simulink model "TDoFs_mass_CL_Trajopt"  (R2022b)
settings: Solver=FixedStepAuto  StartTime=0.0  StopTime=10.0  FixedStep=0.0001  RelTol=1e-3
settings Model: Creator=Taehoon Kim  LastModifiedBy=User
settings ModelReferenceCC: EnableRefExpFcnMdlSchedulingChecks=on

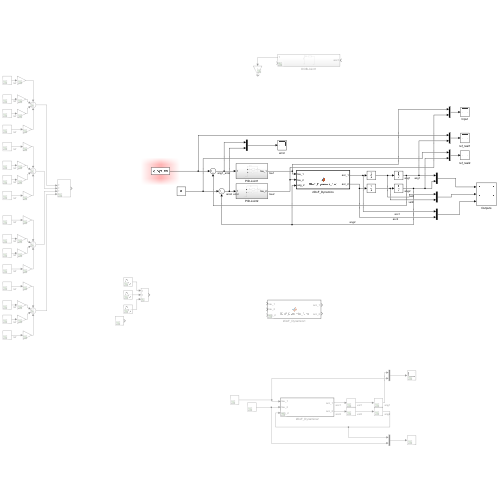
[thumbnail: Simulink's stored preview of the top-level diagram]
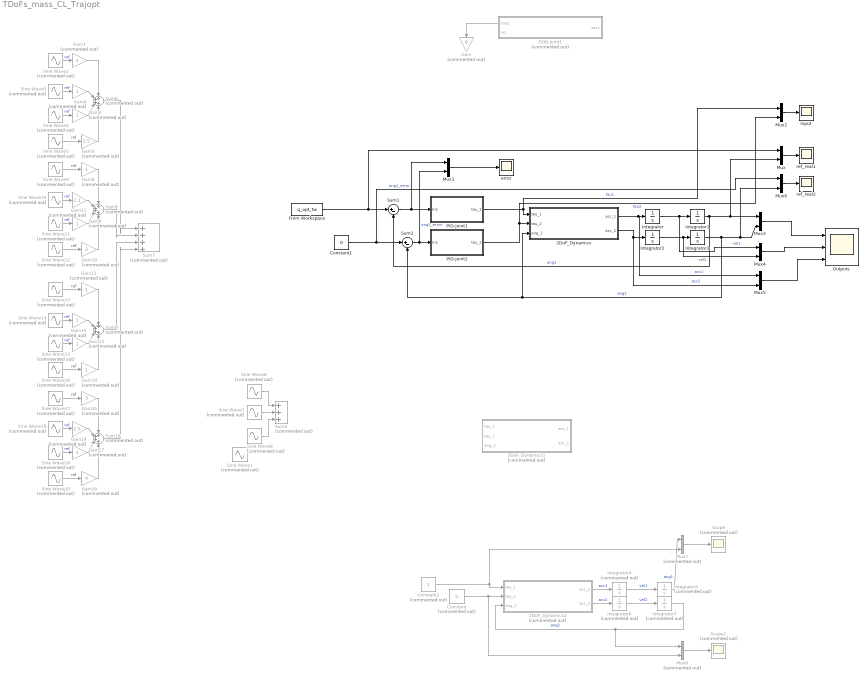
== system TDoFs_mass_CL_Trajopt ==
  2DoF_Dynamics : MATLAB Function  TreatAsAtomicUnit=on
  2DoF_Dynamics1 : MATLAB Function  Commented=on  TreatAsAtomicUnit=on
  2DoF_Dynamics2 : MATLAB Function  Commented=on  TreatAsAtomicUnit=on
  Constant : Constant  Commented=on  Value=0
  Constant1 : Constant  Value=0
  Constant2 : Constant  Commented=on
  DOB-Joint1 : Subsystem  Commented=on
      settings: PortSchema="{\"entries\":[{\"content\":{\"sides\":[{\"content\":{\"connectorIds\":[\"Out1\",\"In1\"]},\"type\":\"ConnectorPlacement.EquallySpacedRectSide\",\"uuid\":\"aed64ee6-890a-40cf-96da-aa5fbca5e20d\"},{\"content\":{\"connectorIds\":[\"In2\"],\"side\":\"RIGHT\"},\"type\":\"ConnectorPlacement.EquallySpacedRectSide\",\"uuid\":\"6cb1d59b-7b2e-4e62-91b9-34dc0f1a000d\"},{\"content\":{\"connectorIds\":[],\"side\":\"TOP\"},\"type\":\"ConnectorPlacement.EquallySpacedRectSide\",\"uuid\":\"fc023f32-e7f5-4e50-b17a-39a9cd0cd429\"},{\"content\":{\"connectorIds\":[],\"side\":\"BOTTOM\"},\"type\":\"ConnectorPlacement.EquallySpacedRectSide\",\"uuid\":\"89f43edb-87a0-44d2-8db4-1bc101ff0a7e\"}]},\"type\":\"ConnectorPlacement.EquallySpacedConnector\",\"uuid\":\"a2668ce1-ca6b-486c-8b99-a7467b774e8d\"}],\"packageUris\":[\"http://schema.mathworks.com/mf0/Connector/R2020b\"],\"version\":\"1.0\"}"
  From Workspace : FromWorkspace  VariableName=q_opt_tw  OutDataTypeStr=double  SampleTime=0.001
  Gain : Gain  Commented=on  Gain=0
  Gain1 : Gain  Commented=on  Gain=5
  Gain10 : Gain  Commented=on  Gain=2
  Gain11 : Gain  Commented=on  Gain=2.1
  Gain{2,4,8..9,12..15,17} (9 alike) : Gain  Commented=on
  Gain16 : Gain  Commented=on  Gain=3
  Gain18 : Gain  Commented=on  Gain=4
  Gain19 : Gain  Commented=on  Gain=2.5
  Gain3 : Gain  Commented=on  Gain=1.5
  Input : Scope
  Integrator{,1..3} (4 alike) : Integrator
  Integrator{4..7} (4 alike) : Integrator  Commented=on
  Mux{,1..6} (7 alike) : Mux  Inputs=2
  Mux7 : Mux  Commented=on  Inputs=2
  Mux8 : Mux  Commented=on  Inputs=2
  Outputs : Scope  NumInputPorts=3
  PID-Joint1 : Subsystem
  PID-Joint2 : Subsystem
  Scope : Scope  Commented=on
  Scope1 : Scope  Commented=on
  Sine Wave1 : Sin  Commented=on  Amplitude=30*(pi/180)  Frequency=2*pi*0.5  SampleTime=0
  Sine Wave10 : Sin  Commented=on  Amplitude=1*(pi/180)  Frequency=0.6*2*pi  SampleTime=0
  Sine Wave11 : Sin  Commented=on  Amplitude=2.1*(pi/180)  Frequency=0.7*2*pi  SampleTime=0
  Sine Wave12 : Sin  Commented=on  Amplitude=2.2*(pi/180)  Frequency=0.8*2*pi  SampleTime=0
  Sine Wave13 : Sin  Commented=on  Amplitude=2*(pi/180)  Frequency=0.9*2*pi  SampleTime=0
  Sine Wave14 : Sin  Commented=on  Amplitude=1.9*(pi/180)  Frequency=1*2*pi  SampleTime=0
  Sine Wave15 : Sin  Commented=on  Amplitude=1.8*(pi/180)  Frequency=1.1*2*pi  SampleTime=0
  Sine Wave16 : Sin  Commented=on  Amplitude=1.7*(pi/180)  Frequency=1.2*2*pi  SampleTime=0
  Sine Wave17 : Sin  Commented=on  Amplitude=1.6*(pi/180)  Frequency=1.3*2*pi  SampleTime=0
  Sine Wave18 : Sin  Commented=on  Amplitude=1.5*(pi/180)  Frequency=1.4*2*pi  SampleTime=0
  Sine Wave19 : Sin  Commented=on  Amplitude=1.3*(pi/180)  Frequency=1.5*2*pi  SampleTime=0
  Sine Wave2 : Sin  Commented=on  Amplitude=1*(pi/180)  Frequency=0.1*2*pi  SampleTime=0
  Sine Wave20 : Sin  Commented=on  Amplitude=1.2*(pi/180)  Frequency=1.5*2*pi  SampleTime=0
  Sine Wave3 : Sin  Commented=on  Amplitude=1.1*(pi/180)  Frequency=0.2*2*pi  SampleTime=0
  Sine Wave4 : Sin  Commented=on  Amplitude=2.4*(pi/180)  Frequency=0.3*2*pi  SampleTime=0
  Sine Wave5 : Sin  Commented=on  Amplitude=2.5*(pi/180)  Frequency=0.4*2*pi  SampleTime=0
  Sine Wave6 : Sin  Commented=on  Amplitude=10*(pi/180)  Frequency=1*2*pi  SampleTime=0
  Sine Wave7 : Sin  Commented=on  Amplitude=20*(pi/180)  Frequency=0.8*2*pi  SampleTime=0
  Sine Wave8 : Sin  Commented=on  Amplitude=2*(pi/180)  Frequency=0.5*2*pi  SampleTime=0
  Sine Wave9 : Sin  Commented=on  Amplitude=2.3*(pi/180)  Frequency=0.5*2*pi  SampleTime=0
  Sum1 : Sum  Inputs=|+-
  Sum{6,8..10} (4 alike) : Sum  Commented=on  Inputs=++++
  Sum2 : Sum  Inputs=|+-
  Sum4 : Sum  Commented=on  Inputs=+++
  Sum7 : Sum  Commented=on  Inputs=|++++
  error : Scope
  ref_real1 : Scope
  ref_real2 : Scope
  wires:
  Integrator1/1 -> Mux/2, Mux3/1, Sum1/2  "ang1"
  Integrator/1 -> Integrator1/1, Mux4/1  "vel1"
  Mux/1 -> ref_real1/1
  Sum1/1 -> Mux1/1, PID-Joint1/1(In1)  "ang1_error"
  PID-Joint1/1(tau_1) -> 2DoF_Dynamics/1(tau_1), Mux2/1  "tau1"
  PID-Joint2/1(tau_2) -> 2DoF_Dynamics/2(tau_2), Mux2/2  "tau2"
  Sum2/1 -> Mux1/2, PID-Joint2/1(In1)  "ang2_error"
  Mux1/1 -> error/1
  Mux2/1 -> Input/1
  2DoF_Dynamics/2(acc_2) -> Integrator2/1, Mux5/2  "acc2"
  Integrator2/1 -> Integrator3/1, Mux4/2  "vel2"
  Integrator3/1 -> Sum2/2, 2DoF_Dynamics/3(ang_2), Mux6/2, Mux3/2  "ang2"
  Mux3/1 -> Outputs/1
  Mux4/1 -> Outputs/2
  2DoF_Dynamics/1(acc_1) -> Mux5/1, Integrator/1  "acc1"
  Mux5/1 -> Outputs/3
  Mux6/1 -> ref_real2/1
  Constant2/1 -> 2DoF_Dynamics2/1(tau_1), Mux7/2
  Constant/1 -> Mux8/2, 2DoF_Dynamics2/2(tau_2)
  2DoF_Dynamics2/1(acc_1) -> Integrator4/1  "acc1"
  Integrator4/1 -> Integrator5/1  "vel1"
  2DoF_Dynamics2/2(acc_2) -> Integrator6/1  "acc2"
  Integrator6/1 -> Integrator7/1  "vel2"
  Integrator7/1 -> Mux8/1, 2DoF_Dynamics2/3(ang_2)  "ang2"
  Integrator5/1 -> Mux7/1  "ang1"
  Mux7/1 -> Scope/1
  Mux8/1 -> Scope1/1
  DOB-Joint1/1(Out1) -> Gain/1
  Sum8/1 -> Sum7/2
  Sine Wave13/1 -> Gain12/1  "ref"
  Sine Wave15/1 -> Gain13/1  "ref"
  Gain15/1 -> Sum9/2
  Gain9/1 -> Sum8/3
  Sine Wave19/1 -> Gain17/1  "ref"
  Gain11/1 -> Sum8/2
  Sum9/1 -> Sum7/3
  Gain14/1 -> Sum9/4
  Sine Wave12/1 -> Gain10/1  "ref"
  Sine Wave20/1 -> Gain18/1  "ref"
  Gain10/1 -> Sum8/4
  Gain3/1 -> Sum6/4
  Sine Wave14/1 -> Gain15/1  "ref"
  Gain18/1 -> Sum10/4
  Gain16/1 -> Sum10/1
  Gain17/1 -> Sum10/3
  Sine Wave10/1 -> Gain11/1  "ref"
  Sum10/1 -> Sum7/4
  Gain2/1 -> Sum6/3
  Sine Wave18/1 -> Gain19/1  "ref"
  Gain4/1 -> Sum6/2
  Sine Wave17/1 -> Gain16/1  "ref"
  Gain19/1 -> Sum10/2
  Gain13/1 -> Sum9/3
  Sine Wave3/1 -> Gain4/1  "ref"
  Sine Wave11/1 -> Gain9/1  "ref"
  Gain12/1 -> Sum9/1
  Sine Wave16/1 -> Gain14/1  "ref"
  Sine Wave4/1 -> Gain2/1  "ref"
  Gain8/1 -> Sum8/1
  Sum6/1 -> Sum7/1
  Sine Wave9/1 -> Gain8/1  "ref"
  Sine Wave5/1 -> Gain3/1  "ref"
  Gain1/1 -> Sum6/1
  Sine Wave2/1 -> Gain1/1  "ref"
  From Workspace/1 -> Mux/1, Sum1/1
  Sine Wave6/1 -> Sum4/1
  Sine Wave8/1 -> Sum4/3
  Sine Wave7/1 -> Sum4/2
  Constant1/1 -> Mux6/1, Sum2/1

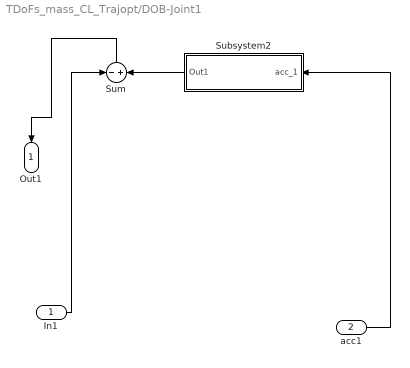
== system TDoFs_mass_CL_Trajopt/DOB-Joint1 ==
  In1 : Inport
  acc1 : Inport  Port=2
  Subsystem2 : Subsystem
  Sum : Sum  Inputs=-+
  Out1 : Outport
  wires:
  In1/1 -> Sum/1
  acc1/1 -> Subsystem2/1(acc_1)
  Subsystem2/1(Out1) -> Sum/2
  Sum/1 -> Out1/1

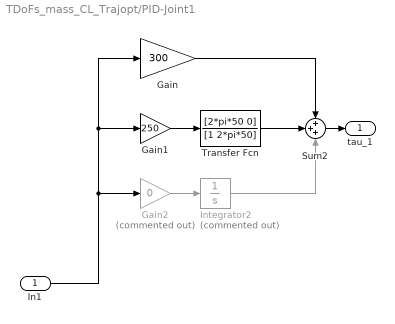
== system TDoFs_mass_CL_Trajopt/PID-Joint1 ==
  In1 : Inport
  Gain : Gain  Gain=300
  Gain1 : Gain  Gain=250
  Gain2 : Gain  Commented=on  Gain=0
  Integrator2 : Integrator  Commented=on
  Sum2 : Sum  Inputs=+++
  Transfer Fcn : TransferFcn  Numerator=[2*pi*50 0]  Denominator=[1 2*pi*50]
  tau_1 : Outport
  wires:
  Gain1/1 -> Transfer Fcn/1
  Gain/1 -> Sum2/1
  Integrator2/1 -> Sum2/3
  In1/1 -> Gain2/1, Gain/1, Gain1/1
  Transfer Fcn/1 -> Sum2/2
  Gain2/1 -> Integrator2/1
  Sum2/1 -> tau_1/1

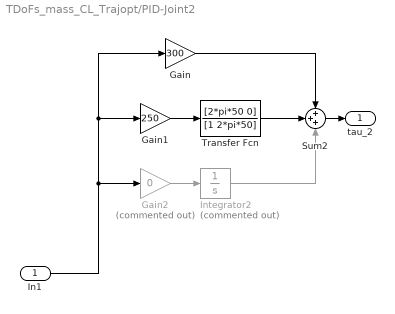
== system TDoFs_mass_CL_Trajopt/PID-Joint2 ==
  In1 : Inport
  Gain : Gain  Gain=300
  Gain1 : Gain  Gain=250
  Gain2 : Gain  Commented=on  Gain=0
  Integrator2 : Integrator  Commented=on
  Sum2 : Sum  Inputs=+++
  Transfer Fcn : TransferFcn  Numerator=[2*pi*50 0]  Denominator=[1 2*pi*50]
  tau_2 : Outport
  wires:
  Sum2/1 -> tau_2/1
  Gain2/1 -> Integrator2/1
  Transfer Fcn/1 -> Sum2/2
  In1/1 -> Gain1/1, Gain/1, Gain2/1
  Integrator2/1 -> Sum2/3
  Gain/1 -> Sum2/1
  Gain1/1 -> Transfer Fcn/1

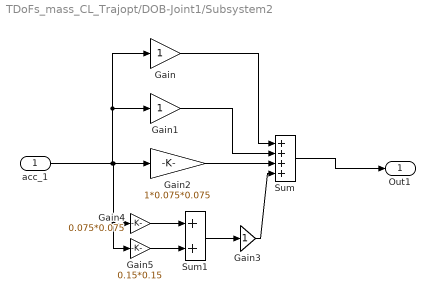
== system TDoFs_mass_CL_Trajopt/DOB-Joint1/Subsystem2 ==
  acc_1 : Inport
  Gain : Gain
  Gain1 : Gain
  Gain2 : Gain  Gain=1*0.075*0.075
  Gain3 : Gain
  Gain4 : Gain  Gain=0.075*0.075
  Gain5 : Gain  Gain=0.15*0.15
  Sum : Sum  Inputs=++++
  Sum1 : Sum
  Out1 : Outport
  wires:
  Sum/1 -> Out1/1
  Gain2/1 -> Sum/3
  Gain1/1 -> Sum/2
  Gain/1 -> Sum/1
  acc_1/1 -> Gain/1, Gain1/1, Gain5/1, Gain4/1, Gain2/1
  Gain3/1 -> Sum/4
  Sum1/1 -> Gain3/1
  Gain4/1 -> Sum1/1
  Gain5/1 -> Sum1/2

== matlab function TDoFs_mass_CL_Trajopt/2DoF_Dynamics1 ==
  data: tau_1 input; acc_1 output; tau_2 input; ang_2 input; acc_2 output
function [acc_1, acc_2] = TDoF_Dynamics_func(tau_1, tau_2, ang_2)
    % Parameters
    J1 = 1;
    J2 = 1;
    l1 = 0.15;
    m2 = 1;
    d1 = 0.075;
    d2 = 0.075;
    
    D = (J2+m2*d2^2)*(J1+J2+m2*d1^2+m2*(2*l1*d2*cos(ang_2)+l1^2+d2^2))-(J2+m2*(l1*d2*cos(ang_2)+d2^2))^2;
    
    acc_1 = ((J2+m2*d2^2)*tau_1+(-J2-m2*(l1*d2*cos(ang_2)+d2^2))*tau_2)/D;
    acc_2 = ((-J2-m2*(l1*d2*cos(ang_2)+d2^2))*tau_1+(J1+J2+m2*d1^2+m2*(2*l1*d2*cos(ang_2)+l1^2+d2^2))*tau_2)/D;
end

== matlab function TDoFs_mass_CL_Trajopt/2DoF_Dynamics ==
  data: tau_1 input; acc_1 output; tau_2 input; ang_2 input; acc_2 output
function [acc_1, acc_2] = TDoF_Dynamics_func(tau_1, tau_2, ang_2)
    % Parameters
    J1 = 1;
    J2 = 1;
    l1 = 0.15;
    m2 = 1;
    d1 = 0.075;
    d2 = 0.075;
    
    D = (J2+m2*d2^2)*(J1+J2+m2*d1^2+m2*(2*l1*d2*cos(ang_2)+l1^2+d2^2))-(J2+m2*(l1*d2*cos(ang_2)+d2^2))^2;
    
    acc_1 = ((J2+m2*d2^2)*tau_1+(-J2-m2*(l1*d2*cos(ang_2)+d2^2))*tau_2)/D;
    acc_2 = ((-J2-m2*(l1*d2*cos(ang_2)+d2^2))*tau_1+(J1+J2+m2*d1^2+m2*(2*l1*d2*cos(ang_2)+l1^2+d2^2))*tau_2)/D;
end

== matlab function TDoFs_mass_CL_Trajopt/2DoF_Dynamics2 ==
  data: tau_1 input; acc_1 output; tau_2 input; ang_2 input; acc_2 output
function [acc_1, acc_2] = TDoF_Dynamics_func(tau_1, tau_2, ang_2)
    % Parameters
    J1 = 1;
    J2 = 1;
    m2 = 1;

    l1 = 0.15;
    d2 = 0.075;
    
    D = J2*(J1*J2+m2*l1^2+2*m2*l1*d2*cos(ang_2))-(J2+m2*l1*d2*cos(ang_2))^2;
    
    acc_1 = (J2*tau_1+(-J2-m2*l1*d2*cos(ang_2))*tau_2)/D;
    acc_2 = ((-J2-m2*l1*d2*cos(ang_2))*tau_1+(J1*J2+m2*l1^2*d2*cos(ang_2))*tau_2)/D;
end
